simulink model "MPPT_ripplecorr"  (Simulink 6.6)
settings: Solver=ode3  StartTime=0.0  StopTime=6  FixedStep=1e-3  RelTol=1e-3
InitFcn:
  | % Ponto de linearização
  | D = 0.5;
  | L = 0.1;
  | C = 0.01;
  | R = 10;
  | Vo = 24;
  | Leq = L/(1-D)^2;
  | N = 1/(1-D);
undefined symbols (not defined in the file): magnitude
libraries: simulink x4, powerlib_extras x1
settings Model: Creator=Luigi2  LastModifiedBy=Batlab

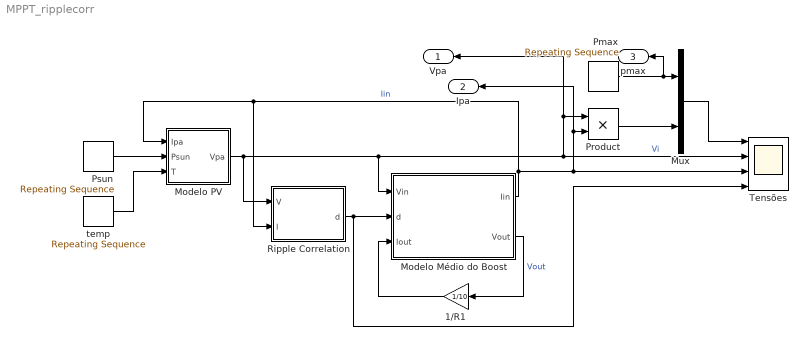
== system MPPT_ripplecorr ==
  1/R1 : Gain  Orientation=left  Gain=1/10
  Modelo Médio do Boost : Subsystem  mask(Modelo de Pequenos Sinais do Boost){L=0.1, Iini=0, C=0.01, Vini=24}
      mask prompts: L "Indutância"; Iini "Corrente inicial"; C "Capacitância"; Vini "Tensão inicial"
      mask help:
      | São entradas do bloco:
      | Vin: Tensão de entrada
      | Iout: Corrente de saída
      | d: ciclo de trabalho
      |
      | São saídas do bloco:
      | Vout: Tensão de saída
      | Iin: Corrente de entrada
      |
      | Devem ser especificados a indutância, a capacitância e os seus valores iniciais para a utilização do modelo.
  Modelo PV : Subsystem
  Mux : Mux  Inputs=2
  Pmax : simulink/Sources/Repeating Sequence  SystemSampleTime=-1  rep_seq_t=[0 2 2 4 4 6]  rep_seq_y=[98.6721 98.6721 187.4175 187.4175 98.6721 98.6721]
  Product : Product  RndMeth=Zero
  Psun : simulink/Sources/Repeating Sequence  SystemSampleTime=-1  rep_seq_t=[0 2 2 4 4 6]  rep_seq_y=[500 500 1000 1000 500 500]
  Ripple Correlation : Subsystem
  Tensões : Scope  NumInputPorts=4
      settings: TimeRange=6  YMin=-50~0~-2~0  YMax=250~40~10~0.8
  temp : simulink/Sources/Repeating Sequence  SystemSampleTime=-1  rep_seq_t=[0 2 2 4 4 6]  rep_seq_y=[25 25 40 40 25 25]
  Vpa : Outport  Orientation=left
  Ipa : Outport  Orientation=left  Port=2
  pmax : Outport  Orientation=left  Port=3
  wires:
  Modelo PV/1(Vpa) -> Modelo Médio do Boost/1(Vin), Tensões/2, Product/1, Vpa/1, Ripple Correlation/1(V)  "Vi"
  Modelo Médio do Boost/2(Vout) -> 1/R1/1  "Vout"
  1/R1/1 -> Modelo Médio do Boost/3(Iout)
  Modelo Médio do Boost/1(Iin) -> Tensões/3, Product/2, Ipa/1, Modelo PV/1(Ipa), Ripple Correlation/2(I)  "Iin"
  Ripple Correlation/1(d) -> Modelo Médio do Boost/2(d), Tensões/4
  Product/1 -> Mux/2
  Psun/1 -> Modelo PV/2(Psun)
  Pmax/1 -> Mux/1, pmax/1
  Mux/1 -> Tensões/1
  temp/1 -> Modelo PV/3(T)

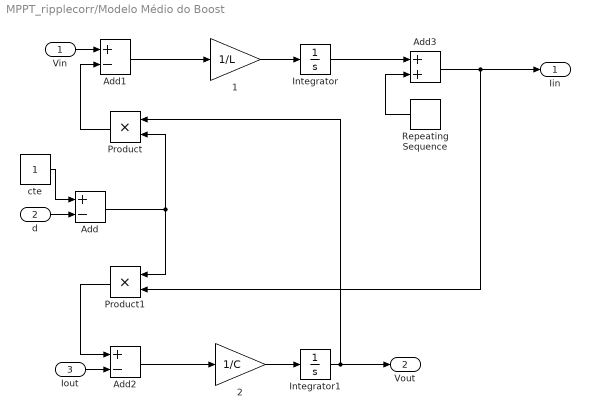
== system MPPT_ripplecorr/Modelo Médio do Boost ==
  Vin : Inport
  d : Inport  Port=2
  Iout : Inport  Port=3
  1 : Gain  Gain=1/L
  2 : Gain  Gain=1/C
  Add : Sum  Inputs=+-  OutScaling=2^-10
  Add1 : Sum  Inputs=+-  OutScaling=2^-10
  Add2 : Sum  Inputs=+-  OutScaling=2^-10
  Add3 : Sum  OutScaling=2^-10
  Integrator : Integrator  InitialCondition=Iini
  Integrator1 : Integrator  InitialCondition=Vini
  Product : Product  Orientation=left  RndMeth=Zero
  Product1 : Product  Orientation=left  RndMeth=Zero
  Repeating Sequence : simulink/Sources/Repeating Sequence  Orientation=left  SystemSampleTime=-1  rep_seq_t=[0 0.5/100 1/100]  rep_seq_y=[-1 1 -1]
  cte : Constant
  Iin : Outport
  Vout : Outport  Port=2
  wires:
  Iout/1 -> Add2/2
  d/1 -> Add/2
  Vin/1 -> Add1/1
  Integrator1/1 -> Product/1, Vout/1
  2/1 -> Integrator1/1
  1/1 -> Integrator/1
  Add2/1 -> 2/1
  Product1/1 -> Add2/1
  Add1/1 -> 1/1
  Add/1 -> Product1/1, Product/2
  Product/1 -> Add1/2
  cte/1 -> Add/1
  Integrator/1 -> Add3/1
  Repeating Sequence/1 -> Add3/2
  Add3/1 -> Product1/2, Iin/1

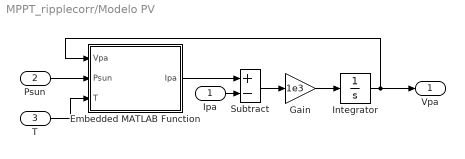
== system MPPT_ripplecorr/Modelo PV ==
  Ipa : Inport
  Psun : Inport  Port=2
  T : Inport  Port=3
  Embedded MATLAB Function : Stateflow chart
  Gain : Gain  Gain=1e3
  Integrator : Integrator  LimitOutput=on  LowerSaturationLimit=0
  Subtract : Sum  Inputs=+-  OutScaling=2^-10
  Vpa : Outport
  wires:
  Psun/1 -> Embedded MATLAB Function/2(Psun)
  T/1 -> Embedded MATLAB Function/3(T)
  Embedded MATLAB Function/1(Ipa) -> Subtract/1
  Subtract/1 -> Gain/1
  Integrator/1 -> Embedded MATLAB Function/1(Vpa), Vpa/1
  Ipa/1 -> Subtract/2
  Gain/1 -> Integrator/1

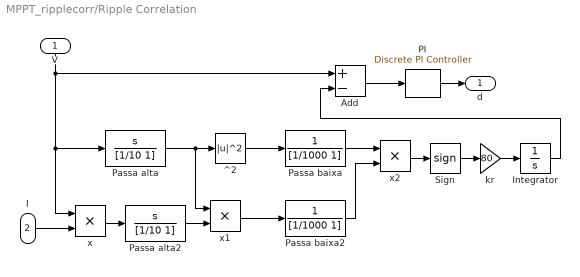
== system MPPT_ripplecorr/Ripple Correlation ==
  V : Inport  Orientation=down
  I : Inport  Port=2
  Add : Sum  Inputs=+-  OutScaling=2^-10
  Integrator : Integrator
  PI : powerlib_extras/Discrete  Control Blocks/Discrete PI Controller  DialogController=POWERSYS.PowerSysDialog  SystemSampleTime=-1  Kp=0.02  Ki=0  Par_Limits=[0.9 0]  Init=0  Ts=1e-3
  Passa alta : TransferFcn  Numerator=[1 0]  Denominator=[1/10 1]
  Passa alta2 : TransferFcn  Numerator=[1 0]  Denominator=[1/10 1]
  Passa baixa : TransferFcn  Denominator=[1/1000 1]
  Passa baixa2 : TransferFcn  Denominator=[1/1000 1]
  Sign : Signum
  ^2 : Math  Operator=magnitude^2  SaturateOnIntegerOverflow=on
  kr : Gain  Gain=80
  x : Product  RndMeth=Zero
  x1 : Product  RndMeth=Zero
  x2 : Product  RndMeth=Zero
  d : Outport
  wires:
  Add/1 -> PI/1
  PI/1 -> d/1
  V/1 -> Passa alta/1, x/1, Add/1
  I/1 -> x/2
  x/1 -> Passa alta2/1
  Passa alta/1 -> x1/1, ^2/1
  Passa alta2/1 -> x1/2
  x1/1 -> Passa baixa2/1
  Passa baixa/1 -> x2/1
  Passa baixa2/1 -> x2/2
  x2/1 -> Sign/1
  Sign/1 -> kr/1
  kr/1 -> Integrator/1
  ^2/1 -> Passa baixa/1
  Integrator/1 -> Add/2

== matlab function Modelo PV/Embedded MATLAB Function ==
  data: Vpa input inherited; Ipa output inherited; Psun input inherited; T input inherited
function Ipa = PV_Array(Vpa, Psun, T) 
Rs = 0.005; 
Rp = 7; 
Ms = 1; % Módulos em Série
Mp = 1; % Módulos em Paralelo
Ns = 54; % No. de células
Voc = 32.9/Ns;
Isc = 8.21; 
a = 3.18e-3; 
n = 1.2; 
k = 1.38e-23; 
q = 1.60e-19; 
EG = 1.1; 
Tr = 273 + 25; 
T = 273 + T; 
Vt = n*k*T/q; 
V = Vpa/Ns/Ms; 
Iph = (Isc+a*(T-Tr))*Psun/1000; 
Irr = (Isc-Voc/Rp)/(exp(q*Voc/n/k/Tr)-1); 
Ir = Irr*(T/Tr)^3*exp(q*EG/n/k*(1/Tr-1/T)); 
I = 0; 
for j=1:5; 
I = I-(Iph-I-Ir*(exp((V+I*Rs)/Vt)-1)-(V+I*Rs)/Rp)/...
    (-1-Ir*exp((V+I*Rs)/Vt)*Rs/Vt-Rs/Rp); 
end 
if I<0, I=0; 
end 
Ipa = I*Mp;
